simulink model "FLNN_Aug_PE1"  (R2024a)
settings: Solver=VariableStepAuto  StartTime=0.0  StopTime=15  RelTol=1e-3
settings Model: Creator=erhan  LastModifiedBy=erhan

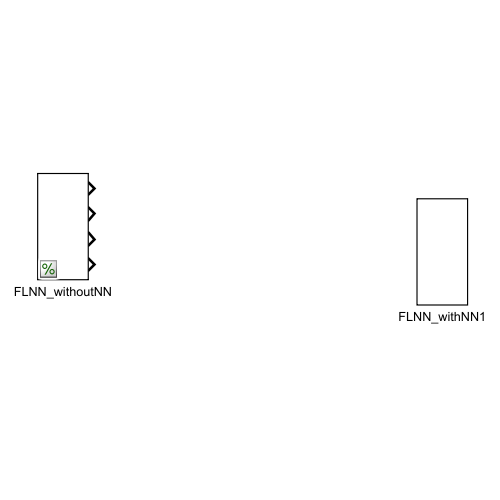
[thumbnail: Simulink's stored preview of the top-level diagram]
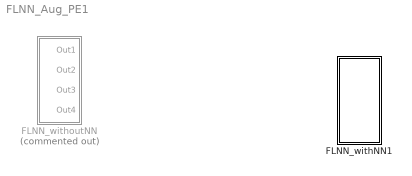
== system FLNN_Aug_PE1 ==
  FLNN_withNN1 : Subsystem
  FLNN_withoutNN : Subsystem  Commented=on

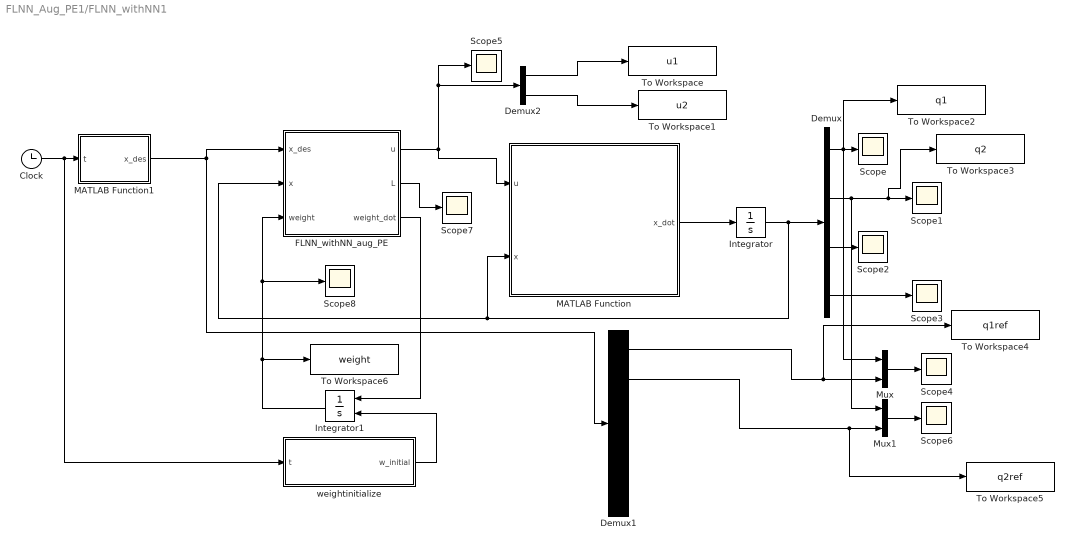
== system FLNN_Aug_PE1/FLNN_withNN1 ==
  Clock : Clock
  Demux : Demux
  Demux1 : Demux  Outputs=6
  Demux2 : Demux  Outputs=2
  FLNN_withNN_aug_PE : MATLAB Function  TreatAsAtomicUnit=on
  Integrator : Integrator  InitialCondition=[0;0;0;0]
  Integrator1 : Integrator  InitialConditionSource=external  InitialCondition=[0;0]
  MATLAB Function : MATLAB Function  TreatAsAtomicUnit=on
  MATLAB Function1 : MATLAB Function  TreatAsAtomicUnit=on
  Mux : Mux  Inputs=2
  Mux1 : Mux  Inputs=2
  Scope{,1..8} (9 alike) : Scope
  To Workspace : ToWorkspace  VariableName=u1  SaveFormat=Timeseries  SampleTime=-1
  To Workspace1 : ToWorkspace  VariableName=u2  SaveFormat=Timeseries  SampleTime=-1
  To Workspace2 : ToWorkspace  VariableName=q1  SaveFormat=Timeseries  SampleTime=-1
  To Workspace3 : ToWorkspace  VariableName=q2  SaveFormat=Timeseries  SampleTime=-1
  To Workspace4 : ToWorkspace  VariableName=q1ref  SaveFormat=Timeseries  SampleTime=-1
  To Workspace5 : ToWorkspace  VariableName=q2ref  SaveFormat=Timeseries  SampleTime=-1
  To Workspace6 : ToWorkspace  VariableName=weight  SaveFormat=Timeseries  SampleTime=-1
  weightinitialize : MATLAB Function  TreatAsAtomicUnit=on
  wires:
  FLNN_withNN_aug_PE/2(L) -> Scope7/1
  Mux1/1 -> Scope6/1
  Demux/4 -> Scope3/1
  Mux/1 -> Scope4/1
  Demux1/1 -> To Workspace4/1, Mux/2
  MATLAB Function1/1(x_des) -> FLNN_withNN_aug_PE/1(x_des), Demux1/1
  Clock/1 -> weightinitialize/1(t), MATLAB Function1/1(t)
  MATLAB Function/1(x_dot) -> Integrator/1
  Demux/3 -> Scope2/1
  Demux/1 -> To Workspace2/1, Scope/1, Mux/1
  Demux/2 -> Mux1/1, To Workspace3/1, Scope1/1
  Demux1/2 -> To Workspace5/1, Mux1/2
  Integrator/1 -> MATLAB Function/2(x), FLNN_withNN_aug_PE/2(x), Demux/1
  FLNN_withNN_aug_PE/3(weight_dot) -> Integrator1/1
  Integrator1/1 -> To Workspace6/1, Scope8/1, FLNN_withNN_aug_PE/3(weight)
  weightinitialize/1(w_initial) -> Integrator1/2
  FLNN_withNN_aug_PE/1(u) -> MATLAB Function/1(u), Demux2/1, Scope5/1
  Demux2/1 -> To Workspace/1
  Demux2/2 -> To Workspace1/1

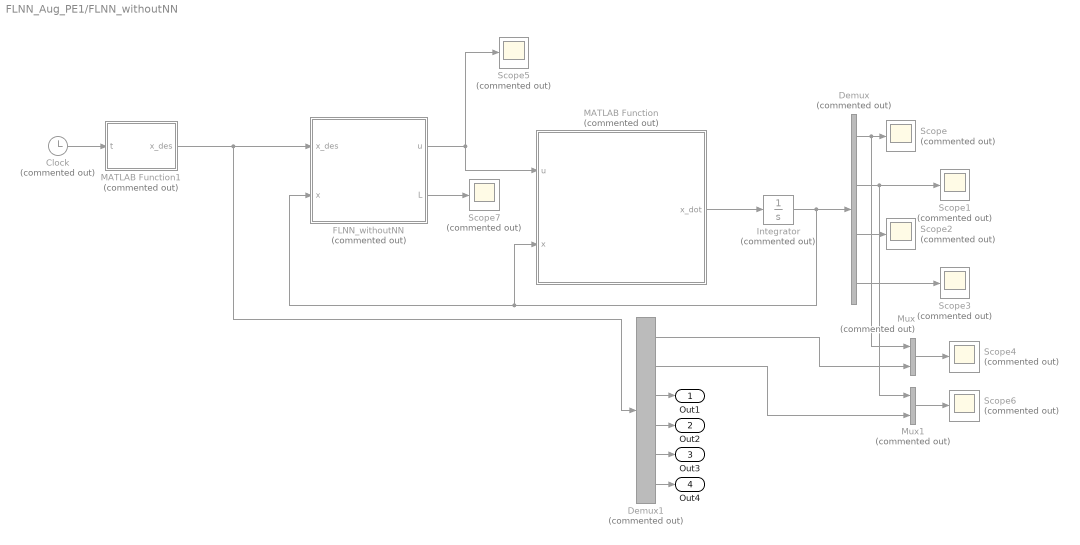
== system FLNN_Aug_PE1/FLNN_withoutNN ==
  Clock : Clock  Commented=on
  Demux : Demux  Commented=on
  Demux1 : Demux  Commented=on  Outputs=6
  FLNN_withoutNN : MATLAB Function  Commented=on  TreatAsAtomicUnit=on
  Integrator : Integrator  Commented=on  InitialCondition=[0;0;0;0]
  MATLAB Function : MATLAB Function  Commented=on  TreatAsAtomicUnit=on
  MATLAB Function1 : MATLAB Function  Commented=on  TreatAsAtomicUnit=on
  Mux : Mux  Commented=on  Inputs=2
  Mux1 : Mux  Commented=on  Inputs=2
  Scope{,1..7} (8 alike) : Scope  Commented=on
  Out1 : Outport
  Out2 : Outport  Port=2
  Out3 : Outport  Port=3
  Out4 : Outport  Port=4
  wires:
  Integrator/1 -> Demux/1, FLNN_withoutNN/2(x), MATLAB Function/2(x)
  FLNN_withoutNN/1(u) -> MATLAB Function/1(u), Scope5/1
  Demux1/3 -> Out1/1
  Demux1/2 -> Mux1/2
  Demux/2 -> Scope1/1, Mux1/1
  Demux/1 -> Mux/1, Scope/1
  Demux/3 -> Scope2/1
  MATLAB Function/1(x_dot) -> Integrator/1
  Clock/1 -> MATLAB Function1/1(t)
  Demux1/4 -> Out2/1
  MATLAB Function1/1(x_des) -> Demux1/1, FLNN_withoutNN/1(x_des)
  Demux1/1 -> Mux/2
  Mux/1 -> Scope4/1
  Demux/4 -> Scope3/1
  Demux1/5 -> Out3/1
  Mux1/1 -> Scope6/1
  FLNN_withoutNN/2(L) -> Scope7/1
  Demux1/6 -> Out4/1

== matlab function FLNN_Aug_PE1/FLNN_withoutNN/FLNN_withoutNN ==
  data: x_des input; u output; x input; L output
function [u,L] = FLNN_withoutNN(x_des,x)

m1=1;
m2=1;
L1=1;
L2=1;
g=9.81;

Kv = 20*eye(2);
lam = 5*eye(2);
qd = x_des(1:2,1); % angle
qdp = x_des(3:4,1); % velocity
qdpp = x_des(5:6,1); % acceleration
e = qd - [x(1) x(2)]';
ep = qdp - [x(3) x(4)]';
r = ep + lam*e;
u = Kv*r;
L=0.5*r*r';
end

== matlab function FLNN_Aug_PE1/FLNN_withoutNN/MATLAB Function ==
  data: u input; x_dot output; x input
function x_dot = RobotDynamic(u,x)
% Parametreler
m1=1;
m2=1;
L1=1;
L2=1;
g=9.81;

% --- M (Atalet) Matrisi ---
M11 = (L1^2*m1)/3 + L1^2*m2 + (L2^2*m2)/3 + L1*L2*m2*cos(x(2));
M12 = (L2*m2*(2*L2 + 3*L1*cos(x(2))))/6;
M21 = M12;
M22 = (L2^2*m2)/3;

% --- C (Coriolis/Merkezkaç) Vektörü ---
C1 = -(L1*L2*x(3)*m2*sin(x(2))*(2*x(3) + x(4)))/2;
C2 = (L1*L2*x(3)^2*m2*sin(x(2)))/2;

% --- G (Yerçekimi) Vektörü ---
G1 = (g*(L2*m2*cos(x(1) + x(2)) + L1*m1*cos(x(1)) + 2*L1*m2*cos(x(1))))/2;
G2 = (L2*g*m2*cos(x(1) + x(2)))/2;


% N (Nonlinear Terms)
N1 = G1 + C1;
N2 = G2 + C2;

% --- MATRİS TERSİ (Inverse Matrix) HESABI ---
% Determinant
det = M11*M22 - M12*M21;

% HATA BURADAYDI (Düzeltildi)
MI11 = M22/det;
MI12 = -M12/det;
MI21 = -M21/det;  % Eksikti, eklendi.
MI22 = M11/det;   % MI11 yerine MI22 yazildi.

% Giriş Torkları
tau1 = u(1);
tau2 = u(2);

% --- İVMELERİN HESAPLANMASI ---
% Denklem: ddq = inv(M) * (tau - N)
% q(3) -> ddq1
% q(4) -> ddq2

q = zeros(4,1);
q(1) = x(3); % dq1
q(2) = x(4); % dq2

% Matris çarpımı (Manuel):
% ddq1 = MI11*(tau1 - N1) + MI12*(tau2 - N2)
q(3) = MI11*(tau1 - N1) + MI12*(tau2 - N2);

% ddq2 = MI21*(tau1 - N1) + MI22*(tau2 - N2)
q(4) = MI21*(tau1 - N1) + MI22*(tau2 - N2);

x_dot = q;
end

== matlab function FLNN_Aug_PE1/FLNN_withoutNN/MATLAB Function1 ==
  data: t input; x_des output
function x_des = ref(t)


period = 2;
amp1 = 0.1;
amp2 = 0.1;
fact = 2*pi/period;
sinf = sin(fact*t);
cosf = cos(fact*t);
qd = [amp1*sinf amp2*cosf];
qdp = fact*[amp1*cosf -amp2*sinf];
qdpp = -fact^2*qd;
x_des = [qd qdp qdpp]';

end

== matlab function FLNN_Aug_PE1/FLNN_withNN1/FLNN_withNN_aug_PE ==
  data: x_des input; u output; x input; L output; weight input; weight_dot output
function [u,L,weight_dot] = FLNN_withNN_aug_PE(x_des,x,weight)

g=9.81;

Kv =150*eye(2);
lam = 20*eye(2);
qd = x_des(1:2,1); % angle
qdp = x_des(3:4,1); % velocity
qdpp = x_des(5:6,1); % acceleration
e = qd - [x(1) x(2)]';
ep = qdp - [x(3) x(4)]';
r = ep + lam*e;
zeta1 = qdpp + lam*ep;
zeta2 = qdp + lam*e;
%%%%%%%%%% FLNN APP
H=4;
K=2;
w = weight;
x_m_q = [zeta1'.*1 , zeta1'.*sin(x(1:2)'), zeta1'.*cos(x(1:2)')];
x_v_m = [zeta2'.*sin(x(1:2)').*x(3:4)', zeta2'.*cos(x(1:2)').*x(3:4)'];
x_g_q = [cos(x(1:2)'), sin(x(1:2)'), sin(x(1:2)').*cos(x(1:2)'), cos(x(1:2)').*cos(x(1:2)')];
x_f_qd = [x(3:4)' , sign(x(3:4)')];


% x_m_q = [zeta1'.*1 , zeta1'.*sin(x(1:2)')];
% x_v_m = [zeta2'.*sin(x(1:2)').*x(3:4)'];
% x_g_q = [cos(x(1:2)'), sin(x(1:2)'), cos(x(1:2)').*cos(x(1:2)')];
% x_f_qd = [x(3:4)'];

phi_x=zeros(H,1);

phi_x(1,1) = sum(x_m_q);
phi_x(2,1) = sum(x_v_m);
phi_x(3,1) = sum(x_g_q);
phi_x(4,1) = sum(x_f_qd);

tau = zeros(K,1);


for k = 1: 1 : K
    cont_int = 0;

    for h = 1:1:H
        cont_int = cont_int+w(h,k)*phi_x(h,1);
    end
    tau(k) = cont_int;
end


    

%%% learning phase

w_dot = zeros(size(w));
F = 50; %% learning rate
kappa = 50;


for k =1 : 1:K
    for h = 1:1:H
        w_dot(h,k) = F*phi_x(h,1)*r(k)-kappa*F*norm(r)*w(h,k);

    end
end

weight_dot = w_dot;
u = tau +  Kv*r;

L = 0.5*r'*r;


end

== matlab function FLNN_Aug_PE1/FLNN_withNN1/MATLAB Function ==
  data: u input; x_dot output; x input
function x_dot = RobotDynamic(u,x)
% Parametreler
m1=0.8;
m2=2.3;
L1=1;
L2=1;
g=9.81;

% --- M (Atalet) Matrisi ---
M11 = (L1^2*m1)/3 + L1^2*m2 + (L2^2*m2)/3 + L1*L2*m2*cos(x(2));
M12 = (L2*m2*(2*L2 + 3*L1*cos(x(2))))/6;
M21 = M12;
M22 = (L2^2*m2)/3;

% --- C (Coriolis/Merkezkaç) Vektörü ---
C1 = -(L1*L2*x(3)*m2*sin(x(2))*(2*x(3) + x(4)))/2;
C2 = (L1*L2*x(3)^2*m2*sin(x(2)))/2;

% --- G (Yerçekimi) Vektörü ---
G1 = (g*(L2*m2*cos(x(1) + x(2)) + L1*m1*cos(x(1)) + 2*L1*m2*cos(x(1))))/2;
G2 = (L2*g*m2*cos(x(1) + x(2)))/2;


% N (Nonlinear Terms)
N1 = G1 + C1;
N2 = G2 + C2;

% --- MATRİS TERSİ (Inverse Matrix) HESABI ---
% Determinant
det = M11*M22 - M12*M21;

% HATA BURADAYDI (Düzeltildi)
MI11 = M22/det;
MI12 = -M12/det;
MI21 = -M21/det;  % Eksikti, eklendi.
MI22 = M11/det;   % MI11 yerine MI22 yazildi.

% Giriş Torkları
tau1 = u(1);
tau2 = u(2);

% --- İVMELERİN HESAPLANMASI ---
% Denklem: ddq = inv(M) * (tau - N)
% q(3) -> ddq1
% q(4) -> ddq2

q = zeros(4,1);
q(1) = x(3); % dq1
q(2) = x(4); % dq2

% Matris çarpımı (Manuel):
% ddq1 = MI11*(tau1 - N1) + MI12*(tau2 - N2)
q(3) = MI11*(tau1 - N1) + MI12*(tau2 - N2);

% ddq2 = MI21*(tau1 - N1) + MI22*(tau2 - N2)
q(4) = MI21*(tau1 - N1) + MI22*(tau2 - N2);

x_dot = q;
end

== matlab function FLNN_Aug_PE1/FLNN_withNN1/MATLAB Function1 ==
  data: t input; x_des output
function x_des = ref(t)


period = 2;
amp1 = 0.1;
amp2 = 0.1;
fact = 2*pi/period;
sinf = sin(fact*t);
cosf = cos(fact*t);
qd = [amp1*sinf amp2*cosf];
qdp = fact*[amp1*cosf -amp2*sinf];
qdpp = -fact^2*qd;
x_des = [qd qdp qdpp]';

end

== matlab function FLNN_Aug_PE1/FLNN_withNN1/weightinitialize ==
  data: t input; w_initial output
function w_initial = weightinitialize(t)

H=4;
K=2;
w=zeros(H,K);
w_initial = w;

end
